simulink model "integral"  (R2023a)
settings: Solver=VariableStepAuto  StartTime=0.0  StopTime=40  RelTol=1e-3
values from neighbouring files (symbols this model uses):
  A = [-4.2386 -0.2026 0.7193 ... (first row only)    [D_stability.m]    (also in Hurwitz_Detectability.m = [-0.0558 -0.9968 0.0802 0.0415; hurwitz_Stabilizability.m = [-1 0 1 1 0 0 -1 2; hurwitz_stability.m = [-0.5 1 0 0 0; schur_stability.m = [-0.5 2 0)
  B = [1 0 0 0 ... (first row only)    [hurwitz_Stabilizability.m]
  C = [0 1 0 0 ... (first row only)    [Hurwitz_Detectability.m]
  H = Ka(size(A,1)+1:end)    [integral.m]
  K = -(1/2)*B'*inv(value(P))    [hurwitz_Stabilizability.m]    (also in integral.m = Ka(1:size(A,1)))
undefined symbols (not defined in the file or in its folder): D
settings Model: Creator=juan  LastModifiedBy=juan

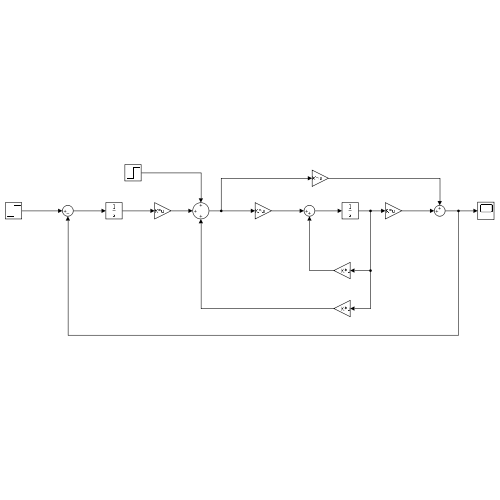
[thumbnail: Simulink's stored preview of the top-level diagram]
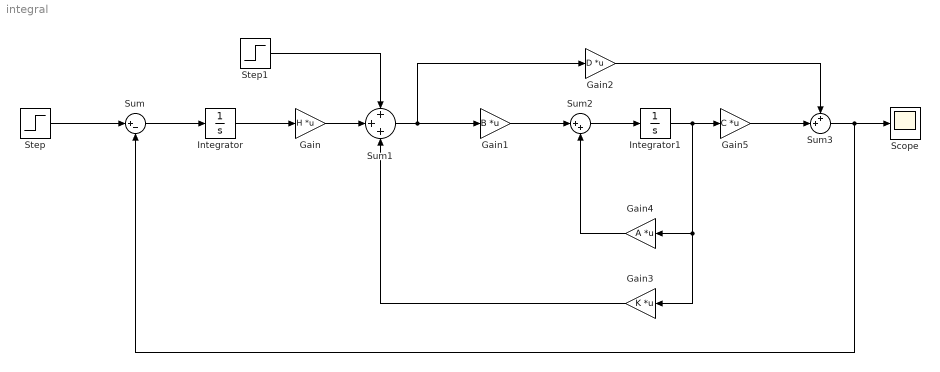
== system integral ==
  Gain : Gain  Gain=H  Multiplication=Matrix(K*u)
  Gain1 : Gain  Gain=B  Multiplication=Matrix(K*u)
  Gain2 : Gain  Gain=D  Multiplication=Matrix(K*u)
  Gain3 : Gain  Gain=K  Multiplication=Matrix(K*u)
  Gain4 : Gain  Gain=A  Multiplication=Matrix(K*u)
  Gain5 : Gain  Gain=C  Multiplication=Matrix(K*u)
  Integrator : Integrator
  Integrator1 : Integrator
  Scope : Scope
  Step : Step  SampleTime=0
  Step1 : Step  Time=20  SampleTime=0
  Sum : Sum  Inputs=|+-
  Sum1 : Sum  Inputs=+++
  Sum2 : Sum  Inputs=|++
  Sum3 : Sum  Inputs=++|
  wires:
  Step/1 -> Sum/1
  Sum/1 -> Integrator/1
  Integrator/1 -> Gain/1
  Sum1/1 -> Gain2/1, Gain1/1
  Gain1/1 -> Sum2/1
  Sum2/1 -> Integrator1/1
  Gain4/1 -> Sum2/2
  Integrator1/1 -> Gain4/1, Gain3/1, Gain5/1
  Gain5/1 -> Sum3/2
  Gain2/1 -> Sum3/1
  Sum3/1 -> Sum/2, Scope/1
  Gain3/1 -> Sum1/3
  Gain/1 -> Sum1/2
  Step1/1 -> Sum1/1
